simulink model "pwmTriangle"  (R2018b)
settings: Solver=VariableStepAuto  StartTime=0.0  StopTime=0.001  RelTol=1e-3
libraries: simulink x1, powerlib_meascontrol x1
settings Model: Creator=K2  LastModifiedBy=K2

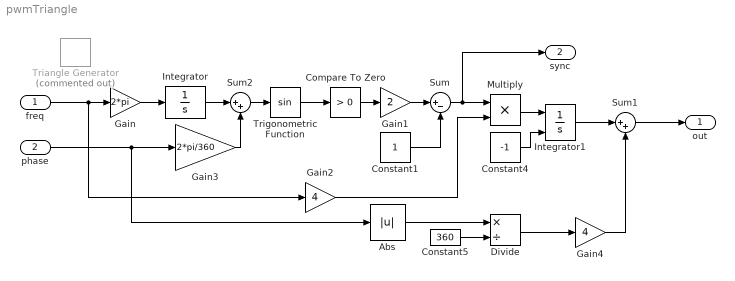
== system pwmTriangle ==
  freq : Inport
  phase : Inport  Port=2
  Abs : Abs
  Compare To Zero : simulink/Logic and Bit Operations/Compare To Zero  relop=>  OutDataTypeStr=boolean
  Constant1 : Constant
  Constant4 : Constant  Value=-1
  Constant5 : Constant  Value=360
  Divide : Product  Inputs=*/
  Gain : Gain  Gain=2*pi
  Gain1 : Gain  Gain=2
  Gain2 : Gain  Gain=4
  Gain3 : Gain  Gain=2*pi/360
  Gain4 : Gain  Gain=4
  Integrator : Integrator
  Integrator1 : Integrator  InitialConditionSource=external
  Multiply : Product
  Sum : Sum  Inputs=|+-
  Sum1 : Sum  Inputs=|++
  Sum2 : Sum  Inputs=|++
  Triangle Generator : powerlib_meascontrol/Pulse & Signal Generators/Triangle Generator  Commented=on  Freq=freq  Phase=167  Ts=0
  Trigonometric Function : Trigonometry
  out : Outport
  sync : Outport  Port=2
  wires:
  freq/1 -> Gain2/1, Gain/1
  Gain/1 -> Integrator/1
  Compare To Zero/1 -> Gain1/1
  Constant1/1 -> Sum/2
  Gain2/1 -> Multiply/2
  Integrator1/1 -> Sum1/1
  Divide/1 -> Gain4/1
  phase/1 -> Gain3/1, Abs/1
  Integrator/1 -> Sum2/1
  Sum2/1 -> Trigonometric Function/1
  Gain3/1 -> Sum2/2
  Gain1/1 -> Sum/1
  Trigonometric Function/1 -> Compare To Zero/1
  Multiply/1 -> Integrator1/1
  Sum/1 -> sync/1, Multiply/1
  Constant5/1 -> Divide/2
  Constant4/1 -> Integrator1/2
  Gain4/1 -> Sum1/2
  Abs/1 -> Divide/1
  Sum1/1 -> out/1
